simulink model "servo_0"  (R2019b)
settings: Solver=VariableStepAuto  StartTime=0.0  StopTime=10.0  RelTol=1e-3
settings Model: Creator=lenovo  LastModifiedBy=lenovo

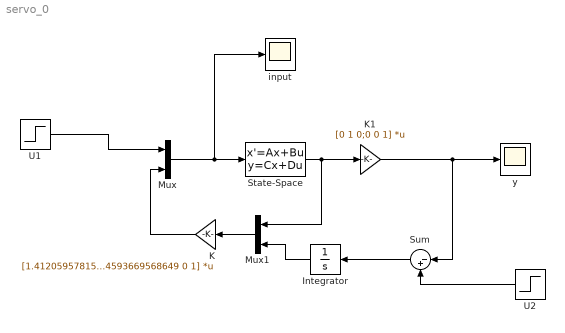
== system servo_0 ==
  Integrator : Integrator
  K : Gain  Gain=|  Multiplication=Matrix(K*u)
      | [1.41205957815341 -3.73155548748854 2.29264297899251
      | 1 0 ;0.383826453251743 0.0266087256763754 1.64593669568649 0 1]
  K1 : Gain  Gain=[0 1 0;0 0 1]  Multiplication=Matrix(K*u)
  Mux : Mux  Inputs=2
  Mux1 : Mux  Inputs=2
  State-Space : StateSpace  A=|  B=|  C=[1 0 0;0 1 0;0 0 1]  D=[0 0 0 0;0 0 0 0;0 0 0 0]  InitialCondition=[1; 100; 200]
      A=|
      | [-1.7 -0.25 0
      |  ;   23 -30 20
      | ;    0 -440 -640]
      B=|
      | [5 0
      |  5 0;-61 0   -61 0
      |   ;0 -550  0 -550]
  Sum : Sum  Inputs=|-+
  U1 : Step  Time=10  After=[-2;5]  SampleTime=0
  U2 : Step  Time=0  After=[100;150]  SampleTime=0
  input : Scope
  y : Scope
  wires:
  State-Space/1 -> Mux1/1, K1/1
  K1/1 -> Sum/1, y/1
  U1/1 -> Mux/1
  K/1 -> Mux/2
  Mux1/1 -> K/1
  U2/1 -> Sum/2
  Sum/1 -> Integrator/1
  Integrator/1 -> Mux1/2
  Mux/1 -> input/1, State-Space/1
